simulink model "Tire1_basic03"  (R2022a)
settings: Solver=VariableStepAuto  StartTime=0.0  StopTime=100  RelTol=1e-3
values from neighbouring files (symbols this model uses):
  Tire_A = 84e-4    (= 0.0084)    [TireParam.m]
  Tire_alpha = -0.003    [TireParam.m]
  Tire_B = 6.2e-4    (= 0.00062)    [TireParam.m]
  Tire_beta = 0.97    [TireParam.m]
  Tire_C = 1.6e-4    (= 0.00016)    [TireParam.m]
  Tire_EffMass = 1/0.4^2    (= 6.25)    [TireParam.m]
  Tire_MagicB = 10    [TireParam.m]
  Tire_MagicC = 1.9    [TireParam.m]
  Tire_MagicD = 0.9    [TireParam.m]
  Tire_MagicE = 0.97    [TireParam.m]
  Tire_pressure = 250e3    (= 250000)    [TireParam.m]
  Tire_R = 0.4    [TireParam.m]
libraries: fl_lib x7, nesl_utility x6, sdl_lib x2
settings Model: Creator=amyyang  LastModifiedBy=amyyang
settings SolverCC: AlgebraicLoopSolver=TrustRegion
settings DebuggingCC: UnconnectedInputMsg=warning  UnconnectedOutputMsg=warning  UnconnectedLineMsg=warning  SFMachineParentedDataDiag=warning
settings RTWCC: DLArmComputeVersion=19.05
settings SimscapeCC: SimscapeLogType=local  SimscapeLogToSDI=on  SimscapeLogLimitData=off

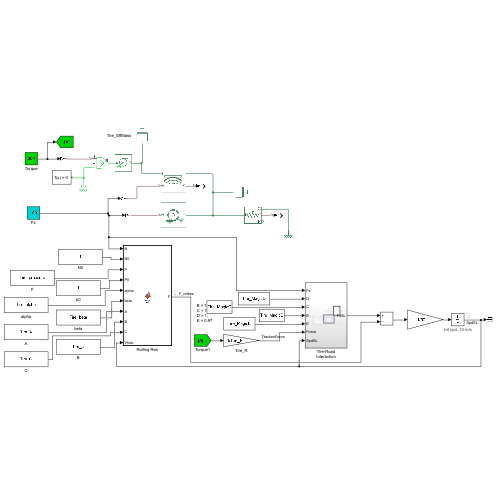
[thumbnail: Simulink's stored preview of the top-level diagram]
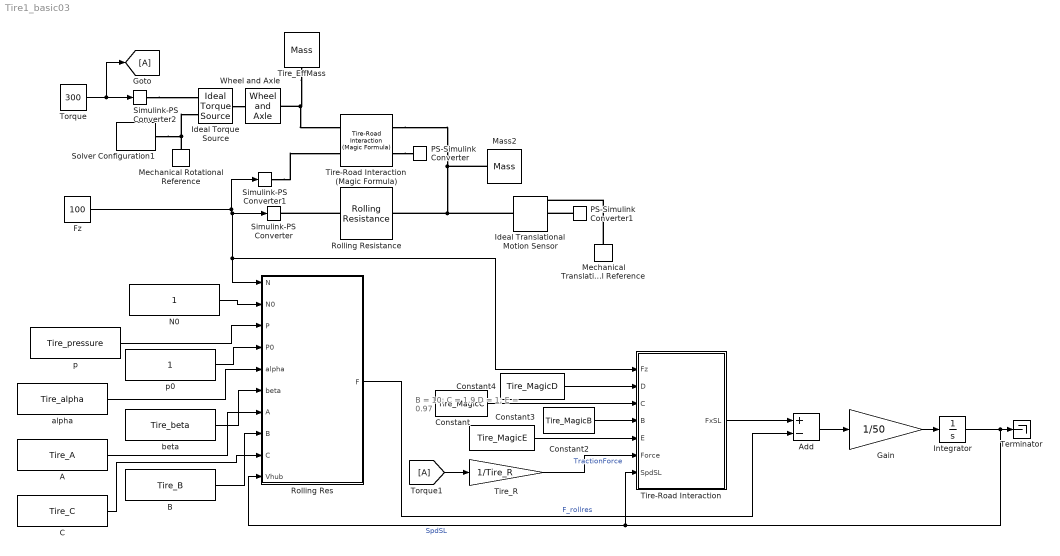
== system Tire1_basic03 ==
  note: B = 10;
      | C = 1.9
      | D = 1;
      | E = 0.97
  A : Constant  Value=Tire_A
  Add : Sum  Inputs=+-
  B : Constant  Value=Tire_B
  C : Constant  Value=Tire_C
  Constant : Constant  Value=Tire_MagicC
  Constant2 : Constant  Value=Tire_MagicB
  Constant3 : Constant  Value=Tire_MagicE
  Constant4 : Constant  Value=Tire_MagicD
  Fz : Constant  Value=100
  Gain : Gain  Gain=1/50
  Goto : Goto
  Ideal Torque Source : fl_lib/Mechanical/Mechanical Sources/Ideal Torque Source
      settings: SourceProductBaseCode=PW,SS,VE
  Ideal Translational Motion Sensor : fl_lib/Mechanical/Mechanical Sensors/Ideal Translational Motion Sensor  offset=0 m
      settings: SourceProductBaseCode=PW,SS,VE
  Integrator : Integrator  InitialCondition=10
      settings: AttributesFormatString=init spd: %<InitialCondition> m/s
  Mass2 : fl_lib/Mechanical/Translational Elements/Mass  mass=50 kg  num_ports=foundation.enum.numPorts2.one  v_specify=on  v_priority=High  v=10 m/s  v_nominal_specify=off  v_nominal_unit=m/s  v_nominal_value=1  f_specify=off  f_priority=None  f=0 N  f_nominal_specify=off  f_nominal_unit=N  f_nominal_value=1
      settings: SourceProductBaseCode=PW,SS,VE  LogSimulationData=on
  Mechanical Rotational Reference : fl_lib/Mechanical/Rotational Elements/Mechanical Rotational Reference
      settings: SourceProductBaseCode=PW,SS,VE
  Mechanical Translational Reference : fl_lib/Mechanical/Translational Elements/Mechanical Translational Reference
      settings: SourceProductBaseCode=PW,SS,VE
  N0 : Constant
  PS-Simulink Converter : nesl_utility/PS-Simulink Converter  PhysicalDomain=network_engine_domain  SubClassName=ps_output  LeftPortType=input  RightPortType=output  PseudoPeriodic=off  Frequencies=[]  VectorFormat=1-D array  Unit=inherit  AffineConversion=off
      settings: SourceProductBaseCode=SS,PW,VE
  PS-Simulink Converter1 : nesl_utility/PS-Simulink Converter  PhysicalDomain=network_engine_domain  SubClassName=ps_output  LeftPortType=input  RightPortType=output  PseudoPeriodic=off  Frequencies=[]  VectorFormat=1-D array  Unit=inherit  AffineConversion=off
      settings: SourceProductBaseCode=SS,PW,VE
  Rolling Res : MATLAB Function  TreatAsAtomicUnit=on
  Rolling Resistance : sdl_lib/Tires & Vehicles/Tire Subcomponents/Rolling Resistance  model=2  coeff=0.015  p_tire=Tire_pressure Pa  alpha=Tire_alpha  beta=Tire_beta  coeff_a=Tire_A  coeff_b=Tire_B s/m  coeff_c=Tire_C s^2/m^2  v_thr=0.001 m/s
      settings: SourceProductBaseCode=LD  LogSimulationData=on  InternalSimscapePortConfiguration="{\"Bottom\":[],\"Left\":[{\"id\":\"N\",\"label\":\"N\",\"type\":\"input\"}],\"Right\":[{\"id\":\"H\",\"label\":\"H\",\"type\":\"foundation.mechanical.translational.translational\"}],\"Top\":[]}"
  Simulink-PS Converter : nesl_utility/Simulink-PS Converter  PhysicalDomain=network_engine_domain  SubClassName=ps_input  LeftPortType=input  RightPortType=output  PseudoPeriodic=off  Frequencies=[]  NoiseDistribution=none  NoiseParameters=[]  Unit=N  AffineConversion=off  FilteringAndDerivatives=provide  SimscapeFilterOrder=1  InputFilterTimeConstant=0.001  UdotUserProvided=0
      settings: SourceProductBaseCode=SS,PW,VE
  Simulink-PS Converter1 : nesl_utility/Simulink-PS Converter  PhysicalDomain=network_engine_domain  SubClassName=ps_input  LeftPortType=input  RightPortType=output  PseudoPeriodic=off  Frequencies=[]  NoiseDistribution=none  NoiseParameters=[]  Unit=N  AffineConversion=off  FilteringAndDerivatives=provide  SimscapeFilterOrder=1  InputFilterTimeConstant=0.001  UdotUserProvided=0
      settings: SourceProductBaseCode=SS,PW,VE
  Simulink-PS Converter2 : nesl_utility/Simulink-PS Converter  PhysicalDomain=network_engine_domain  SubClassName=ps_input  LeftPortType=input  RightPortType=output  PseudoPeriodic=off  Frequencies=[]  NoiseDistribution=none  NoiseParameters=[]  Unit=N*m  AffineConversion=off  FilteringAndDerivatives=provide  SimscapeFilterOrder=1  InputFilterTimeConstant=0.001  UdotUserProvided=0
      settings: SourceProductBaseCode=SS,PW,VE
  Solver Configuration1 : nesl_utility/Solver Configuration  PhysicalDomain=network_engine_domain  SubClassName=solver  LeftPortType=input  RightPortType=generic  Tones=[]  Harmonics=[]  SimulateNoise=off  Profile=off  UseLocalSampling=off  EnableSwitchedLinearOptims=on  FrequencyDomain=off  UseCCode=off  RelTol=0.001  AbsTol=1e-06  MinStep=1e-09  ToWorkspace=off  RevertToSquareIcSolve=off  NumHomotopyIterations=100  PhasorMode=off  PhasorModeNumHarmonics=1  IndexReductionMethod=DerivativeReplacement  DoDC=off  ResidualTolerance=1e-09  UseLocalSolver=off  LocalSolverChoice=NE_BACKWARD_EULER_ADVANCER  LocalSolverSampleTime=0.001  DoFixedCost=off  MaxNonlinIter=3  MaxModeIter=2  ComputeImpulses=off  ImpulseIterations=2  LinearAlgebra=auto  LinearAlgebraNumThread=0  EquationFormulation=NE_TIME_EF  DelaysMemoryBudget=1024  AutomaticFiltering=on  FilteringTimeConstant=0.001  PartitionStorageMethod=AS_NEEDED  PartitionMemoryBudget=1024  PartitionMethod=ROBUST
      settings: SourceProductBaseCode=SS,PW,VE
  Terminator : Terminator
  Tire-Road Interaction : Subsystem
  Tire-Road Interaction (Magic Formula) : sdl_lib/Tires & Vehicles/Tire Subcomponents/Tire-Road Interaction (Magic Formula)  parameterization=sdl.enum.magic_tire_model.constant  F_z1=3000 N  F_x1=3500 N  kappa1=10  B_m=Tire_MagicB  C_m=Tire_MagicC  D_m=Tire_MagicD  E_m=Tire_MagicE  fz0=4000 N  p_Cx=1.685  p_Dx=[1.21, -.037]  p_Ex=[.344, .095, -.02, 0]  p_Kx=[21.51, -.163, .245]  p_Hx=[-.002, .002]  p_Vx=[0, 0]  v_tr_thr=0.1 m/s
      settings: SourceProductBaseCode=LD  LogSimulationData=on  InternalSimscapePortConfiguration="{\"Bottom\":[],\"Left\":[{\"id\":\"N\",\"label\":\"N\",\"type\":\"input\"},{\"id\":\"T\",\"label\":\"T\",\"type\":\"foundation.mechanical.translational.translational\"}],\"Right\":[{\"id\":\"S\",\"label\":\"S\",\"type\":\"output\"},{\"id\":\"H\",\"label\":\"H\",\"type\":\"foundation.mechanical.translational.translational\"}],\"Top\":[]}"
  Tire_EffMass : fl_lib/Mechanical/Translational Elements/Mass  mass=Tire_EffMass kg  num_ports=foundation.enum.numPorts2.one  v_specify=off  v_priority=High  v=0 m/s  v_nominal_specify=off  v_nominal_unit=m/s  v_nominal_value=1  f_specify=off  f_priority=None  f=0 N  f_nominal_specify=off  f_nominal_unit=N  f_nominal_value=1
      settings: SourceProductBaseCode=PW,SS,VE
  Tire_R : Gain  Gain=1/Tire_R
  Torque : Constant  Value=300
  Torque1 : From
  Wheel and Axle : fl_lib/Mechanical/Mechanisms/Wheel and Axle  R=Tire_R m  or=1  t_specify=off  t_priority=None  t=0 N*m  t_nominal_specify=off  t_nominal_unit=N*m  t_nominal_value=1  f_specify=off  f_priority=None  f=0 N  f_nominal_specify=off  f_nominal_unit=N  f_nominal_value=1
      settings: SourceProductBaseCode=PW,SS,VE  LogSimulationData=on
  alpha : Constant  Value=Tire_alpha
  beta : Constant  Value=Tire_beta
  p : Constant  Value=Tire_pressure
  p0 : Constant
  wires:
  p/1 -> Rolling Res/3(P)
  p0/1 -> Rolling Res/4(P0)
  alpha/1 -> Rolling Res/5(alpha)
  beta/1 -> Rolling Res/6(beta)
  B/1 -> Rolling Res/8(B)
  C/1 -> Rolling Res/9(C)
  A/1 -> Rolling Res/7(A)
  Rolling Res/1(F) -> Add/2  "F_rollres"
  N0/1 -> Rolling Res/2(N0)
  Torque/1 -> Goto/1, Simulink-PS Converter2/1
  Torque1/1 -> Tire_R/1
  Gain/1 -> Integrator/1
  Fz/1 -> Tire-Road Interaction/1(Fz), Rolling Res/1(N), Simulink-PS Converter/1, Simulink-PS Converter1/1
  Constant4/1 -> Tire-Road Interaction/2(D)
  Constant/1 -> Tire-Road Interaction/3(C)
  Constant2/1 -> Tire-Road Interaction/4(B)
  Constant3/1 -> Tire-Road Interaction/5(E)
  Tire-Road Interaction/1(FxSL) -> Add/1
  Tire_R/1 -> Tire-Road Interaction/6(Force)  "TractionForce"
  Integrator/1 -> Rolling Res/10(Vhub), Tire-Road Interaction/7(SpdSL), Terminator/1  "SpdSL"
  Add/1 -> Gain/1
  connections:
  Rolling Resistance/LConn1 -- Simulink-PS Converter/RConn1
  Mass2/LConn1 -- Tire-Road Interaction (Magic Formula)/RConn2 -- Ideal Translational Motion Sensor/LConn1 -- Rolling Resistance/RConn1
  Tire_EffMass/LConn1 -- Tire-Road Interaction (Magic Formula)/LConn2 -- Wheel and Axle/RConn1
  Tire-Road Interaction (Magic Formula)/RConn1 -- PS-Simulink Converter/LConn1
  Simulink-PS Converter2/RConn1 -- Ideal Torque Source/RConn1
  Simulink-PS Converter1/RConn1 -- Tire-Road Interaction (Magic Formula)/LConn1
  Ideal Torque Source/LConn1 -- Wheel and Axle/LConn1
  Mechanical Rotational Reference/LConn1 -- Solver Configuration1/RConn1 -- Ideal Torque Source/RConn2
  Mechanical Translational Reference/LConn1 -- Ideal Translational Motion Sensor/RConn1
  PS-Simulink Converter1/LConn1 -- Ideal Translational Motion Sensor/RConn2

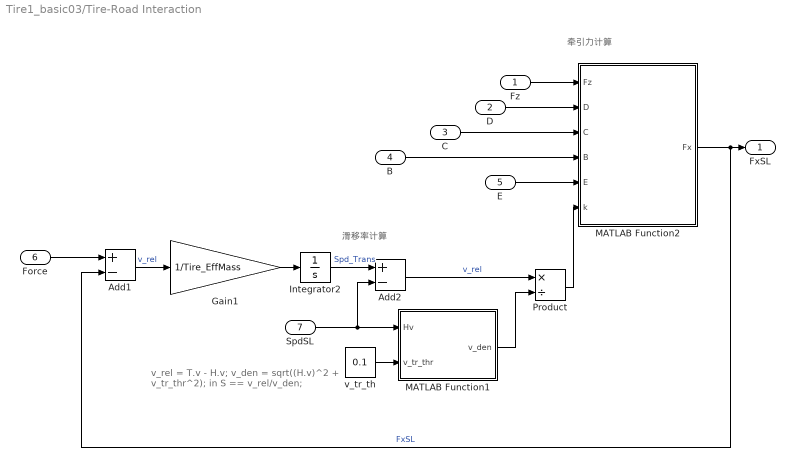
== system Tire1_basic03/Tire-Road Interaction ==
  note: 牵引力计算
  note: 滑移率计算
  note: v_rel = T.v - H.v;
      |         v_den = sqrt((H.v)^2 + v_tr_thr^2);
      |     in
      |         S == v_rel/v_den;
  Fz : Inport
  D : Inport  Port=2
  C : Inport  Port=3
  B : Inport  Port=4
  E : Inport  Port=5
  Force : Inport  Port=6
  SpdSL : Inport  Port=7
  Add1 : Sum  Inputs=+-
  Add2 : Sum  Inputs=+-
  Gain1 : Gain  Gain=1/Tire_EffMass
  Integrator2 : Integrator
  MATLAB Function1 : MATLAB Function  TreatAsAtomicUnit=on
  MATLAB Function2 : MATLAB Function  TreatAsAtomicUnit=on
  Product : Product  Inputs=*/
  v_tr_th : Constant  Value=0.1
  FxSL : Outport
  wires:
  SpdSL/1 -> MATLAB Function1/1(Hv), Add2/2
  Gain1/1 -> Integrator2/1
  v_tr_th/1 -> MATLAB Function1/2(v_tr_thr)
  MATLAB Function1/1(v_den) -> Product/2
  Fz/1 -> MATLAB Function2/1(Fz)
  Add1/1 -> Gain1/1  "v_rel"
  Add2/1 -> Product/1  "v_rel"
  Product/1 -> MATLAB Function2/6(k)
  MATLAB Function2/1(Fx) -> FxSL/1, Add1/2  "FxSL"
  Integrator2/1 -> Add2/1  "Spd_Trans"
  D/1 -> MATLAB Function2/2(D)
  Force/1 -> Add1/1
  C/1 -> MATLAB Function2/3(C)
  B/1 -> MATLAB Function2/4(B)
  E/1 -> MATLAB Function2/5(E)

== matlab function Tire1_basic03/Tire-Road Interaction/MATLAB Function2 ==
  data: Fz input; D input; C input; B input; E input; Fx output; k input
function Fx = fcn(Fz,D,C,B,E,k)

Fx = Fz * D*sin(C*atan(B*k - E*(B*k - atan(B*k))));
end

== matlab function Tire1_basic03/Rolling Res ==
  data: N input; N0 input; P input; F output; P0 input; alpha input; beta input; A input; B input; C input; Vhub input
function F = fcn(N,N0,P,P0,alpha,beta,A,B,C,Vhub)

F = (P/P0)^alpha * (N/N0)^beta*(A + B*abs(Vhub) + C* Vhub^2);

== matlab function Tire1_basic03/Tire-Road Interaction/MATLAB Function1 ==
  data: Hv input; v_den output; v_tr_thr input
function v_den = fcn(Hv,v_tr_thr)

 v_den = sqrt((Hv)^2 + v_tr_thr^2);
end
